simulink model "TTypeModulation"  (R2023b)
settings: Solver=FixedStepAuto  StartTime=0.0  StopTime=4/ffund  FixedStep=1e-6  MaxStep=1e-7  RelTol=1e-3
InitFcn:
  | fsw=5500;
  | ffund=500;
  | ma=0.5;
libraries: spsTriangleGeneratorLib x2
settings Model: Creator=lbocker  LastModifiedBy=enesa
settings DebuggingCC: SignalInfNanChecking=warning

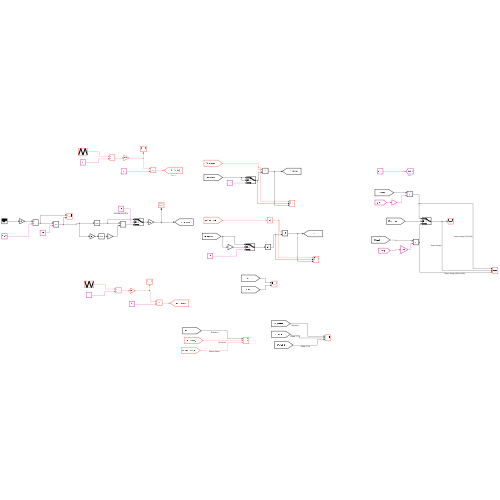
[thumbnail: Simulink's stored preview of the top-level diagram]
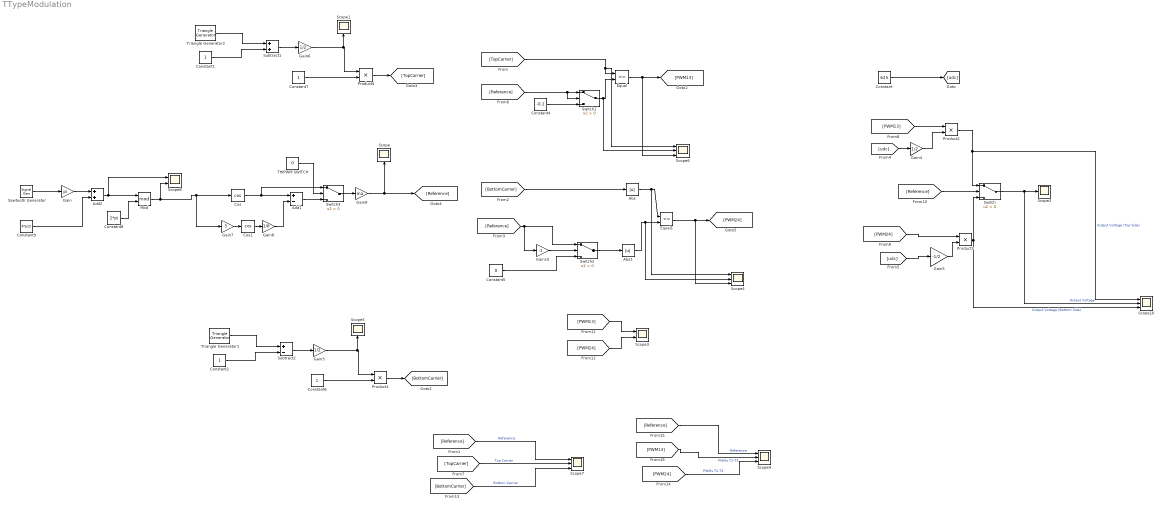
== system TTypeModulation ==
  Abs : Abs  SaturateOnIntegerOverflow=off
  Abs1 : Abs  SaturateOnIntegerOverflow=off
  Add1 : Sum  Inputs=+-
  Add2 : Sum
  Constant : Constant  Value=625
  Constant{1..2,6..7} (4 alike) : Constant
  Constant4 : Constant  Value=-0.1
  Constant5 : Constant  Value=0
  Constant8 : Constant  Value=2*pi
  Constant9 : Constant  Value=3*pi/2
  Cos : Trigonometry  Operator=cos
  Cos1 : Trigonometry  Operator=cos
  Equal : RelationalOperator  Operator=<=  OutDataTypeStr=boolean  RndMeth=Simplest  InputSameDT=off
  Equal1 : RelationalOperator  Operator=<=  OutDataTypeStr=boolean  RndMeth=Simplest  InputSameDT=off
  Gain : Gain  Gain=pi
  Gain10 : Gain  Gain=-1
  Gain3 : Gain  Gain=1/2
  Gain4 : Gain  Gain=1/2
  Gain5 : Gain  Gain=-1/2
  Gain6 : Gain  Gain=1/2
  Gain7 : Gain  Gain=3
  Gain8 : Gain  Gain=1/6
  Gain9 : Gain  Gain=ma
  Mod : Math  Operator=mod
  Product{1..4} (4 alike) : Product
  Sawtooth Generator : SignalGenerator  WaveForm=sawtooth  Frequency=2*pi*ffund  Units=rad/sec
  Scope{,1..2,5} (4 alike) : Scope
  Scope{4,6..7,9..10} (5 alike) : Scope  NumInputPorts=3
  Scope3 : Scope  NumInputPorts=2
  Scope8 : Scope  NumInputPorts=2
  Subtract1 : Sum
  Subtract2 : Sum  Inputs=+-
  Switch{,1..3} (4 alike) : Switch  Criteria=u2 > Threshold  SaturateOnIntegerOverflow=off  InputSameDT=off
  "THIPWM SWITCH " : Constant  Value=0
  Triangle Generator1 : spsTriangleGeneratorLib/Triangle Generator  Freq=fsw*2  Phase=180  Ts=1e-6
  Triangle Generator2 : spsTriangleGeneratorLib/Triangle Generator  Freq=fsw*2  Phase=0  Ts=1e-6
  wires:
  Product3/1 -> Switch/3, Scope10/3  "Output Voltage (Bottom Side)"
  Constant2/1 -> Subtract2/2
  [udc] -> Gain5/1
  Gain4/1 -> Product2/2
  [udc] -> Gain4/1
  Gain5/1 -> Product3/2
  Subtract2/1 -> Gain3/1
  Constant6/1 -> Product1/2
  Constant/1 -> [udc]
  Gain3/1 -> Product1/1, Scope5/1
  Product2/1 -> Scope10/1, Switch/1  "Output Voltage (Top Side)"
  Triangle Generator1/1 -> Subtract2/1
  Switch/1 -> Scope10/2, Scope2/1  "Output Voltage"
  Product1/1 -> [BottomCarrier]
  Product4/1 -> [TopCarrier]
  Constant7/1 -> Product4/2
  Triangle Generator2/1 -> Subtract1/1
  Constant1/1 -> Subtract1/2
  Gain6/1 -> Product4/1, Scope1/1
  Subtract1/1 -> Gain6/1
  [Reference] -> Switch1/2, Switch1/1
  Constant4/1 -> Switch1/3
  [Reference] -> Gain10/1, Switch2/1
  Switch2/1 -> Abs1/1
  Constant5/1 -> Switch2/3
  Gain7/1 -> Cos1/1
  Cos1/1 -> Gain8/1
  Cos/1 -> Switch3/1, Add1/1
  Gain8/1 -> Add1/2
  Add1/1 -> Switch3/3
  Switch3/1 -> Gain9/1
  "THIPWM SWITCH "/1 -> Switch3/2
  Gain9/1 -> [Reference], Scope/1
  Equal/1 -> Scope6/3, [PWM13]
  Equal1/1 -> Scope4/3, [PWM24]
  [PWM13] -> Product2/1
  [PWM24] -> Product3/1
  [Reference] -> Switch/2
  [PWM13] -> Scope3/1
  [PWM24] -> Scope3/2
  Gain10/1 -> Switch2/2
  [TopCarrier] -> Scope6/1, Equal/1
  Switch1/1 -> Scope6/2, Equal/2
  [Reference] -> Scope7/1  "Reference"
  [TopCarrier] -> Scope7/2  "Top Carrier"
  [BottomCarrier] -> Scope7/3  "Bottom Carrier"
  Mod/1 -> Scope8/2, Cos/1, Gain7/1
  Constant8/1 -> Mod/2
  Sawtooth Generator/1 -> Gain/1
  Constant9/1 -> Add2/2
  Add2/1 -> Scope8/1, Mod/1
  Gain/1 -> Add2/1
  [PWM24] -> Scope9/3  "PWMs T2-T4"
  [Reference] -> Scope9/1  "Reference"
  [PWM13] -> Scope9/2  "PWMs T1-T3"
  [BottomCarrier] -> Abs/1
  Abs/1 -> Scope4/1, Equal1/1
  Abs1/1 -> Scope4/2, Equal1/2
